simulink model "drone_spring_2dof_sfun"  (R2025b)
settings: Solver=ode45  StartTime=0.0  StopTime=0.5  MaxStep=2e-4  RelTol=1e-3
settings Model: Creator=seung  LastModifiedBy=seung

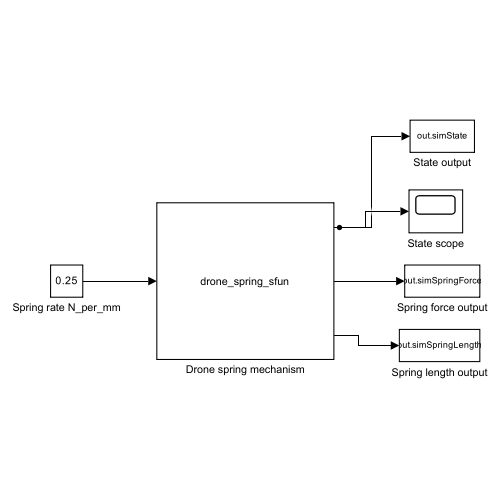
[thumbnail: Simulink's stored preview of the top-level diagram]
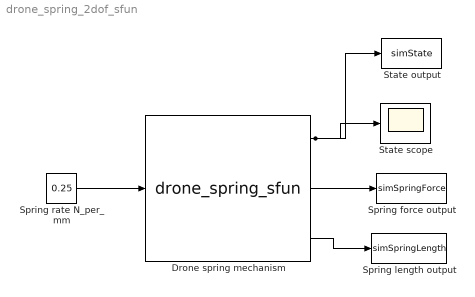
== system drone_spring_2dof_sfun ==
  Drone spring mechanism : M-S-Function  FunctionName=drone_spring_sfun
  Spring force output : ToWorkspace  VariableName=simSpringForce  SaveFormat=Timeseries  SampleTime=-1
  Spring length output : ToWorkspace  VariableName=simSpringLength  SaveFormat=Timeseries  SampleTime=-1
  Spring rate N_per_mm : Constant  Value=0.25
  State output : ToWorkspace  VariableName=simState  SaveFormat=Timeseries  SampleTime=-1
  State scope : Scope
  wires:
  Drone spring mechanism/3 -> Spring length output/1
  Drone spring mechanism/2 -> Spring force output/1
  Spring rate N_per_mm/1 -> Drone spring mechanism/1
  Drone spring mechanism/1 -> State output/1, State scope/1
